simulink model "ELADRC_Model"  (R2020a)
settings: Solver=VariableStepAuto  StartTime=0.0  StopTime=0.01  RelTol=1e-3
settings Model: PacingRate=0.001000  Creator=Bryan  LastModifiedBy=Bryan

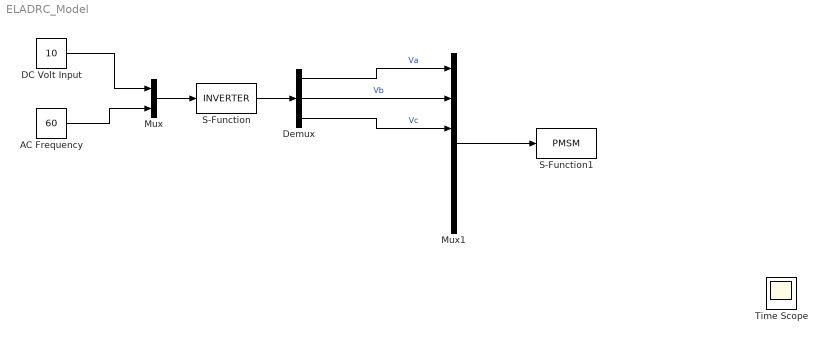
== system ELADRC_Model ==
  AC Frequency : Constant  Value=60
  DC Volt Input : Constant  Value=10
  Demux : Demux  Outputs=3
  Mux : Mux  Inputs=2
  Mux1 : Mux  Inputs=6
  S-Function : S-Function  FunctionName=INVERTER  SFunctionDeploymentMode=off  EnableBusSupport=off
  S-Function1 : S-Function  FunctionName=PMSM  SFunctionDeploymentMode=off  EnableBusSupport=off
  Time Scope : Scope
  wires:
  Mux/1 -> S-Function/1
  DC Volt Input/1 -> Mux/1
  AC Frequency/1 -> Mux/2
  S-Function/1 -> Demux/1
  Demux/2 -> Mux1/2  "Vb"
  Demux/1 -> Mux1/1  "Va"
  Demux/3 -> Mux1/3  "Vc"
  Mux1/1 -> S-Function1/1
